simulink model "Edge_Formation"  (R2025a)
settings: Solver=VariableStepAuto  StartTime=0.0  StopTime=50  RelTol=1e-3
settings Model: Creator=huy01  LastModifiedBy=huy01

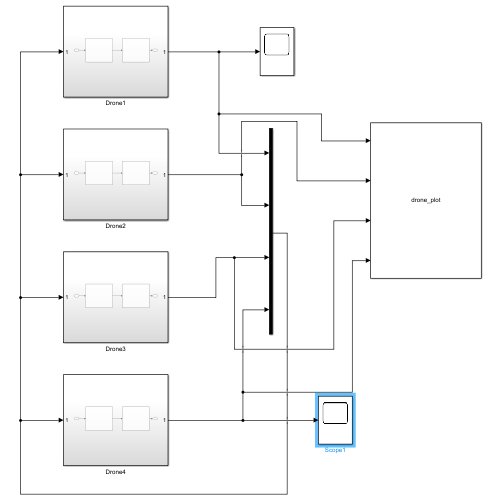
[thumbnail: Simulink's stored preview of the top-level diagram]
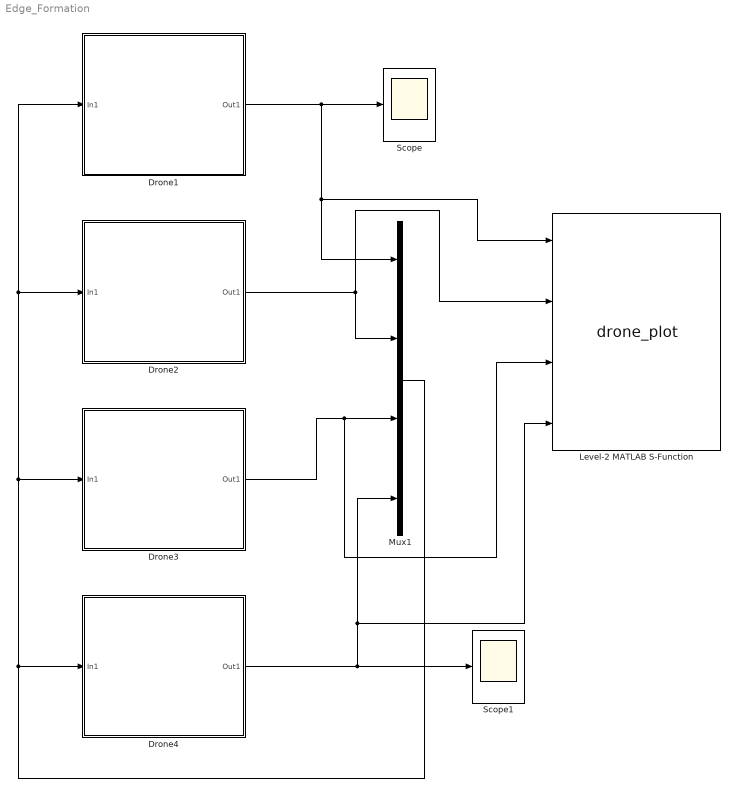
== system Edge_Formation ==
  Drone1 : Subsystem
  Drone2 : Subsystem
  Drone3 : Subsystem
  Drone4 : Subsystem
  Level-2 MATLAB S-Function : M-S-Function  FunctionName=drone_plot
  Mux1 : Mux
  Scope : Scope
      settings: ActiveDisplayYMinimum=-0.84476269505805712  ActiveDisplayYMaximum=7.961335608295844
  Scope1 : Scope
      settings: ActiveDisplayYMinimum=-1  ActiveDisplayYMaximum=1
  wires:
  Drone1/1(Out1) -> Scope/1, Level-2 MATLAB S-Function/1, Mux1/1
  Drone2/1(Out1) -> Mux1/2, Level-2 MATLAB S-Function/2
  Drone3/1(Out1) -> Level-2 MATLAB S-Function/3, Mux1/3
  Drone4/1(Out1) -> Scope1/1, Level-2 MATLAB S-Function/4, Mux1/4
  Mux1/1 -> Drone4/1(In1), Drone3/1(In1), Drone2/1(In1), Drone1/1(In1)

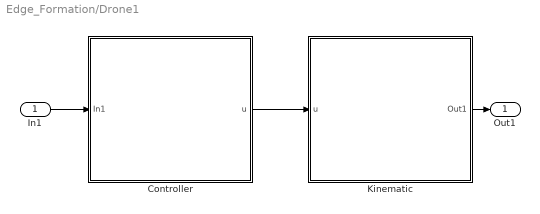
== system Edge_Formation/Drone1 ==
  In1 : Inport
  Controller : Subsystem
  Kinematic : Subsystem
  Out1 : Outport
  wires:
  Controller/1(u) -> Kinematic/1(u)
  Kinematic/1(Out1) -> Out1/1
  In1/1 -> Controller/1(In1)

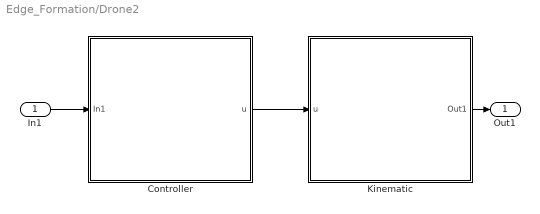
== system Edge_Formation/Drone2 ==
  In1 : Inport
  Controller : Subsystem
  Kinematic : Subsystem
  Out1 : Outport
  wires:
  Controller/1(u) -> Kinematic/1(u)
  Kinematic/1(Out1) -> Out1/1
  In1/1 -> Controller/1(In1)

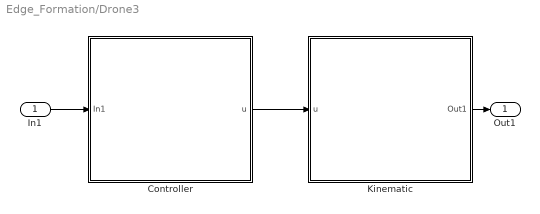
== system Edge_Formation/Drone3 ==
  In1 : Inport
  Controller : Subsystem
  Kinematic : Subsystem
  Out1 : Outport
  wires:
  Controller/1(u) -> Kinematic/1(u)
  Kinematic/1(Out1) -> Out1/1
  In1/1 -> Controller/1(In1)

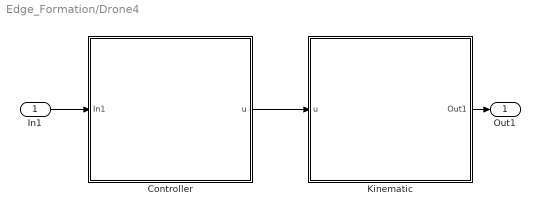
== system Edge_Formation/Drone4 ==
  In1 : Inport
  Controller : Subsystem
  Kinematic : Subsystem
  Out1 : Outport
  wires:
  Controller/1(u) -> Kinematic/1(u)
  Kinematic/1(Out1) -> Out1/1
  In1/1 -> Controller/1(In1)

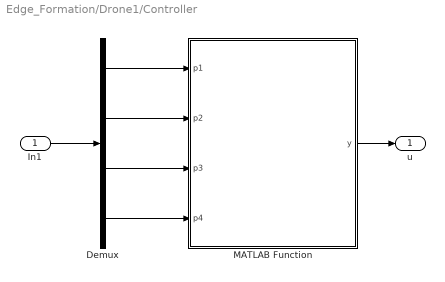
== system Edge_Formation/Drone1/Controller ==
  In1 : Inport
  Demux : Demux
  MATLAB Function : MATLAB Function  TreatAsAtomicUnit=on
  u : Outport
  wires:
  MATLAB Function/1(y) -> u/1
  In1/1 -> Demux/1
  Demux/1 -> MATLAB Function/1(p1)
  Demux/2 -> MATLAB Function/2(p2)
  Demux/3 -> MATLAB Function/3(p3)
  Demux/4 -> MATLAB Function/4(p4)

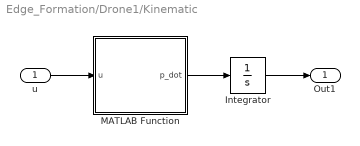
== system Edge_Formation/Drone1/Kinematic ==
  u : Inport
  Integrator : Integrator  InitialCondition=10*rand(3,1)
  MATLAB Function : MATLAB Function  TreatAsAtomicUnit=on
  Out1 : Outport
  wires:
  u/1 -> MATLAB Function/1(u)
  MATLAB Function/1(p_dot) -> Integrator/1
  Integrator/1 -> Out1/1

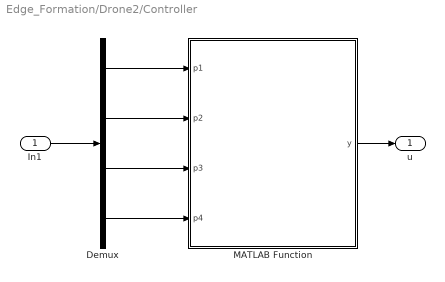
== system Edge_Formation/Drone2/Controller ==
  In1 : Inport
  Demux : Demux
  MATLAB Function : MATLAB Function  TreatAsAtomicUnit=on
  u : Outport
  wires:
  MATLAB Function/1(y) -> u/1
  In1/1 -> Demux/1
  Demux/1 -> MATLAB Function/1(p1)
  Demux/2 -> MATLAB Function/2(p2)
  Demux/3 -> MATLAB Function/3(p3)
  Demux/4 -> MATLAB Function/4(p4)

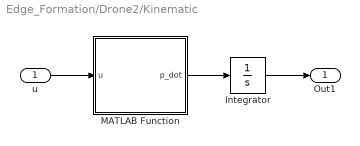
== system Edge_Formation/Drone2/Kinematic ==
  u : Inport
  Integrator : Integrator  InitialCondition=10*rand(3,1)
  MATLAB Function : MATLAB Function  TreatAsAtomicUnit=on
  Out1 : Outport
  wires:
  u/1 -> MATLAB Function/1(u)
  MATLAB Function/1(p_dot) -> Integrator/1
  Integrator/1 -> Out1/1

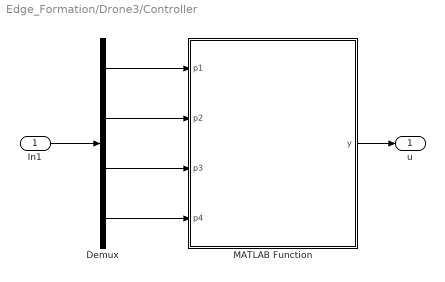
== system Edge_Formation/Drone3/Controller ==
  In1 : Inport
  Demux : Demux
  MATLAB Function : MATLAB Function  TreatAsAtomicUnit=on
  u : Outport
  wires:
  MATLAB Function/1(y) -> u/1
  In1/1 -> Demux/1
  Demux/1 -> MATLAB Function/1(p1)
  Demux/2 -> MATLAB Function/2(p2)
  Demux/3 -> MATLAB Function/3(p3)
  Demux/4 -> MATLAB Function/4(p4)

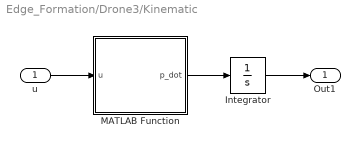
== system Edge_Formation/Drone3/Kinematic ==
  u : Inport
  Integrator : Integrator  InitialCondition=10*rand(3,1)
  MATLAB Function : MATLAB Function  TreatAsAtomicUnit=on
  Out1 : Outport
  wires:
  u/1 -> MATLAB Function/1(u)
  MATLAB Function/1(p_dot) -> Integrator/1
  Integrator/1 -> Out1/1

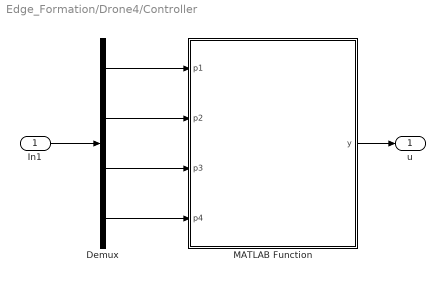
== system Edge_Formation/Drone4/Controller ==
  In1 : Inport
  Demux : Demux
  MATLAB Function : MATLAB Function  TreatAsAtomicUnit=on
  u : Outport
  wires:
  MATLAB Function/1(y) -> u/1
  In1/1 -> Demux/1
  Demux/1 -> MATLAB Function/1(p1)
  Demux/2 -> MATLAB Function/2(p2)
  Demux/3 -> MATLAB Function/3(p3)
  Demux/4 -> MATLAB Function/4(p4)

== system Edge_Formation/Drone4/Kinematic ==
  u : Inport
  Integrator : Integrator  InitialCondition=10*rand(3,1)
  MATLAB Function : MATLAB Function  TreatAsAtomicUnit=on
  Out1 : Outport
  wires:
  u/1 -> MATLAB Function/1(u)
  MATLAB Function/1(p_dot) -> Integrator/1
  Integrator/1 -> Out1/1

== matlab function Edge_Formation/Drone1/Controller/MATLAB Function ==
  data: p1 input; y output; p2 input; p3 input; p4 input
function y = fcn(p1, p2, p3, p4)
    e12 = 3; e13 = 5; e14 = 4; e23 = 4; e24 = 5; e34 = 3;

    y = 0.01*((norm(p2-p1)^2 - e12^2)*(p2-p1) + (norm(p3-p1)^2 - e13^2)*(p3-p1) + (norm(p4-p1)^2 - e14^2)*(p4-p1));

end

== matlab function Edge_Formation/Drone1/Kinematic/MATLAB Function ==
  data: u input; p_dot output
function p_dot = fcn(u)

    p_dot = u;

end

== matlab function Edge_Formation/Drone2/Controller/MATLAB Function ==
  data: p1 input; y output; p2 input; p3 input; p4 input
function y = fcn(p1, p2, p3, p4)
    e12 = 3; e13 = 5; e14 = 4; e23 = 4; e24 = 5; e34 = 3;

    y = 0.01*((norm(p2-p1)^2 - e12^2)*(p1-p2) + (norm(p3-p2)^2 - e23^2)*(p3-p2) + (norm(p4-p2)^2 - e24^2)*(p4-p2));

end

== matlab function Edge_Formation/Drone2/Kinematic/MATLAB Function ==
  data: u input; p_dot output
function p_dot = fcn(u)

    p_dot = u;

end

== matlab function Edge_Formation/Drone3/Controller/MATLAB Function ==
  data: p1 input; y output; p2 input; p3 input; p4 input
function y = fcn(p1, p2, p3, p4)
    e12 = 3; e13 = 5; e14 = 4; e23 = 4; e24 = 5; e34 = 3;

    y = 0.01*((norm(p3-p1)^2 - e13^2)*(p1-p3) + (norm(p3-p2)^2 - e23^2)*(p2-p3) + (norm(p4-p3)^2 - e34^2)*(p4-p3));

end

== matlab function Edge_Formation/Drone3/Kinematic/MATLAB Function ==
  data: u input; p_dot output
function p_dot = fcn(u)

    p_dot = u;

end

== matlab function Edge_Formation/Drone4/Controller/MATLAB Function ==
  data: p1 input; y output; p2 input; p3 input; p4 input
function y = fcn(p1, p2, p3, p4)
    e12 = 3; e13 = 5; e14 = 4; e23 = 4; e24 = 5; e34 = 3;

    y = 0.01*((norm(p4-p1)^2 - e14^2)*(p1-p4) + (norm(p4-p2)^2 - e24^2)*(p2-p4) + (norm(p4-p3)^2 - e34^2)*(p3-p4));

end

== matlab function Edge_Formation/Drone4/Kinematic/MATLAB Function ==
  data: u input; p_dot output
function p_dot = fcn(u)

    p_dot = u;

end
